simulink library "etherlab_lib"  (Simulink 7.4)
settings: Solver=ode45  SolverMode=SingleTasking  StartTime=0.0  StopTime=10.0  RelTol=1e-3
undefined symbols (not defined in the file or in its folder): Address, baumer_ecatencoder, el320x, el500x, el5101, el5101_0010, EL5151, El5152, el515x, ep41xx, ep43xx, rv, x
(part 3 of 3)

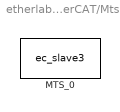
== system etherlab_lib/EtherCAT/Mts ==
  MTS_0 : S-Function  FunctionName=ec_slave3  Parameters=address, rv.SlaveConfig, rv.PortConfig, debug, tsample  SFunctionModules='ecrt_support'  EnableBusSupport=off  mask(MTS R-Series){master=0, index=1, model=1 Magnet, offset=0, invert=off, velocity_output=off, status_output=off, filter=off, tau=[], tsample=0, debug=0}
      mask prompts: index "Slave Index"; model "Device Model"; offset "Output Offset"; invert "Invert Position / Velocity"; velocity_output "Velocity Output"; status_output "Status Output"; filter "Output Filter"; tau "LPF Time Constant [s]"; tsample "Sample Time"
      mask help:
      | MTS R-Series Position Senor
      |
      | Output 1: position vector (magnets 1-5) in meter
      | Optional output 2: speed vector (magnets 1-5) in m/s
      | Optional output 3: status vector (magnets 1-5)
      mask init:
      | masterStr = '';
      | positionStr = '';
      | 
      | [address masterStr positionStr] = ...
      |         getEtherCATAddress(gcb, master, index, tsample);
      | 
      | rv = mts_temposonics(model, offset, filter, tau, ...
      |                      invert, velocity_output, status_output);
      mask Help:
      | This block generically implements the MTS R-Series Position Sensor for various models.
      | <p/>
      | The following Terminals are supported:
      | <center>
      | <table width="80%">
      | <tr><td>1 Magnet</td><td> </td></tr>
      | <tr><td>2 Magnets</td><td> </td></tr>
      | <tr><td>3 Magnets</td><td> </td></tr>
      | <tr><td>4 Magnets</td><td> </td></tr>
      | <tr><td>5 Magnets</td><td> </td></tr>
      | </table>
      | </center>
      | <p/>
      | Choose and set the following options:
      | <h4>Master:</h4>
      | Set the EtherCAT Master of this terminal.
      | 
      | <h4>Slave Index:</h4>
      | Set the EtherCAT slave index. Following address formats are allowed:
      | <ol>
      | <li> Absolute addressing: a scalar number <<b><tt>n</tt></b>> representing the (zero based) absolute position in the bus.
      | <li> SSId addressing: the Secondary Slave (or 'Alias') Addressing has the form <<b><tt>[alias position]</tt></b>> where <b><tt>alias</tt></b> is the Secondary Slave Id of the EtherCAT slave and <b><tt>position</tt></b> is the offset after the slave with the given <b><tt>alias</tt></b>. The SSId has to be preprogrammed into the slave with other service tools (see 'ethercat alias --help').
      | </ol>
      | 
      | <h4>Device Model:</h4>
      | Choose the model at the Indexed position of the master.
      | 
      | <p>
      | Choosing <b>Status Output</b> provides a port of type <tt>uint8_T</tt> where the status is presented. This is only enabled when <b>Vector Output</b> is selected. Terminal input over- and underrange can be detected using this output. See the terminal's documentation.
      | 
      | <h4>Output Filter</h4>
      | When not in <b>Raw</b> mode, the <b>Output Filter</b> checkbox becomes available, allowing the use of an internal low pass filter. Enter the <b>LPF Time Constant</b> for the filter in the field below.
      | <br>For continuous sample time systems (0 in Sample Time), the filter is also continuous. Discrete samples systems (Sample Time > 0) uses an equivalent discrete low pass filter with a similar time constant.
      | 
      | <p>
      | Set the <b>Sample Time</b> for the block. <tt>0</tt> is continuous sample time (runs at the model's base rate). Setting <tt>-1</tt> will try to set the time using back propagation.
      mask StyleString: edit,edit,popup(1 Magnet|2 Magnets|3 Magnets|4 Magnets|5 Magnets),edit,checkbox,checkbox,checkbox,checkbox,edit,edit,edit
      mask CallbackString: |||||||mtsrseries_check('filter');|||
      mask Display: fprintf('MTS R-Series\n%s\n%s Idx:%s',model,masterStr,positionStr);

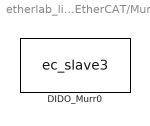
== system etherlab_lib/EtherCAT/Murr ==
  DIDO_Murr0 : S-Function  FunctionName=ec_slave3  Parameters=Address,rv.SlaveConfig,rv.PortConfig,debug,tsample  SFunctionModules='ecrt_support'  EnableBusSupport=off  mask(Murr Impact67 EC){master=0, index=1, model=DI8DO8, vector=on, tsample=0, debug=0}
      mask prompts: index "Slave Index"; model "Device Model"; vector "Vector IO"; tsample "Sample Time (-1 for inherited)"
      mask help:
      | Murr Impact67 EC
      | Digital  IO-Terminal
      mask init:
      | masterStr = '';
      | positionStr = '';
      | [Address masterStr positionStr] = ...
      |     getEtherCATAddress(gcb,master,index,tsample);
      | 
      | rv = get_param(gcbh,'UserData');
      mask Help: web(etherlab_help_path('murr_dio.html'), '-helpbrowser');
      mask StyleString: edit,edit,popup(DI16|DI8DO8|DO16|DO8),checkbox,edit,edit
      mask CallbackString: ||murr_dio('set');|murr_dio('set');||
      mask Display:
      | fprintf('Murr Impact 67 EC\n%s\nM:%s Idx:%s',...
      |     model,masterStr,positionStr)

== system etherlab_lib/EtherCAT/Subsystem ==
